simulink model "simulink_caso4_digital"  (R2023a)
settings: Solver=VariableStepAuto  StartTime=0.0  StopTime=6  MaxStep=0.001  MinStep=0.0001  RelTol=1e-3  EnableMultiTasking=on
undefined symbols (not defined in the file): Ad, Aestd, Bd, Bestd, C, Cestd, D, Destd, K00d, Kd, T, Ts
settings Model: Creator=54115  LastModifiedBy=Agustin
settings SolverCC: AlgebraicLoopSolver=TrustRegion
settings DataIOCC: ReturnWorkspaceOutputs=off
settings OptimizationCC: LifeSpan=inf
settings DebuggingCC: UnconnectedInputMsg=warning  UnconnectedOutputMsg=warning  UnconnectedLineMsg=warning  SFUnexpectedBacktrackingDiag=warning  SFNoUnconditionalDefaultTransitionDiag=warning  ArithmeticOperatorsInVariantConditions=warning
settings ModelReferenceCC: EnableRefExpFcnMdlSchedulingChecks=on
settings SFSimCC: SimUseLocalCustomCode=off  CustomCodeUndefinedFunction=UseInterfaceOnly
settings RTWCC: RTWUseLocalCustomCode=off
settings CodeAppCC: StateflowObjectComments=on
settings GRTTargetCC: TargetLangStandard=C89/C90 (ANSI)
settings ConfigComp: CovMetricSettings=dw  CovSaveCumulativeToWorkspaceVar=on  CovSaveSingleToWorkspaceVar=on  CovExternalEMLEnable=off

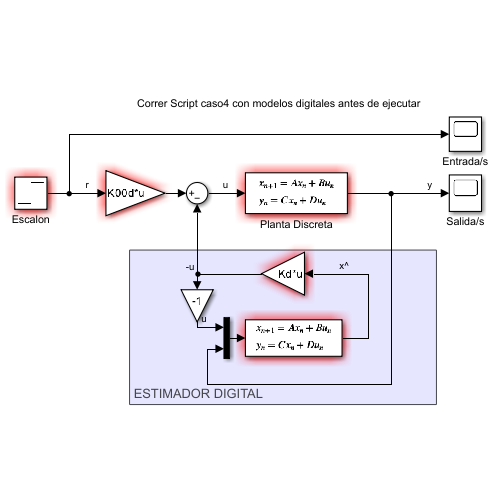
[thumbnail: Simulink's stored preview of the top-level diagram]
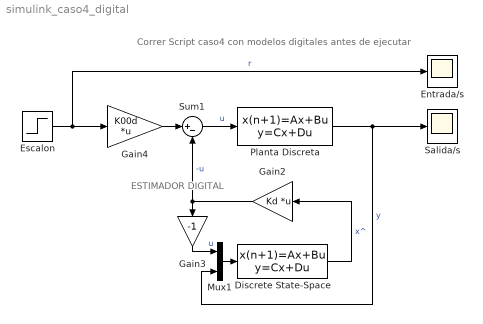
== system simulink_caso4_digital ==
  note: ESTIMADOR DIGITAL
  note: Correr Script caso4 con modelos digitales antes de ejecutar
  Discrete State-Space : DiscreteStateSpace  A=Aestd  B=Bestd  C=Cestd  D=Destd  SampleTime=Ts
  Entrada/s : Scope
  Escalon : Step  Time=0  SampleTime=Ts
  Gain2 : Gain  Gain=Kd  Multiplication=Matrix(K*u)
  Gain3 : Gain  Gain=-1
  Gain4 : Gain  Gain=K00d  Multiplication=Matrix(K*u)
  Mux1 : Mux  Inputs=2
  Planta Discreta : DiscreteStateSpace  A=Ad  B=Bd  C=C  D=D  SampleTime=T
  Salida/s : Scope
  Sum1 : Sum  Inputs=|+-
  wires:
  Discrete State-Space/1 -> Gain2/1  "x^"
  Sum1/1 -> Planta Discreta/1  "u"
  Escalon/1 -> Entrada/s/1, Gain4/1  "r"
  Gain4/1 -> Sum1/1
  Mux1/1 -> Discrete State-Space/1
  Planta Discreta/1 -> Mux1/2, Salida/s/1  "y"
  Gain2/1 -> Gain3/1, Sum1/2  "-u"
  Gain3/1 -> Mux1/1  "u"
